simulink model "Flight_sim"  (R2023b)
settings: Solver=ode45  StartTime=0.0  StopTime=350  RelTol=1e-3
values from neighbouring files (symbols this model uses):
  g = 9.81    [parms.m]
  gam_0 = pi/2    (= 1.57079632679)    [parms.m]
  gam_in = 0.10    (= 0.1)    [parms.m]
  h0 = 0    [parms.m]
  m = 132    [parms.m]
  m_zfw = m_dry+m_pay    (= 6360.7)    [parms.m]
  RE = 6371e3    (= 6371000)    [parms.m]
  t_turn = 30    [parms.m]
  v0 = 0.01    [parms.m]
  x0 = 0    [parms.m]
libraries: slpidlib x1, simulink x1
settings Model: Creator=Legrey  LastModifiedBy=Legrey

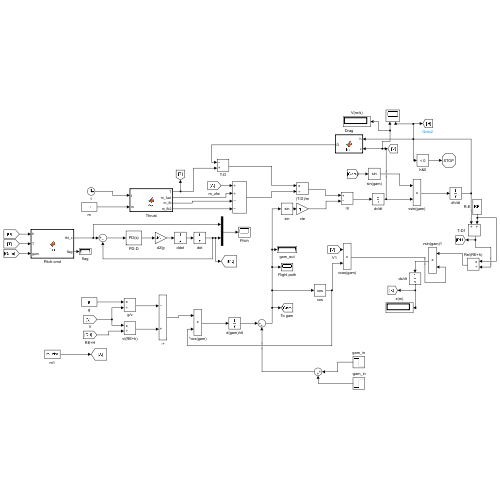
[thumbnail: Simulink's stored preview of the top-level diagram]
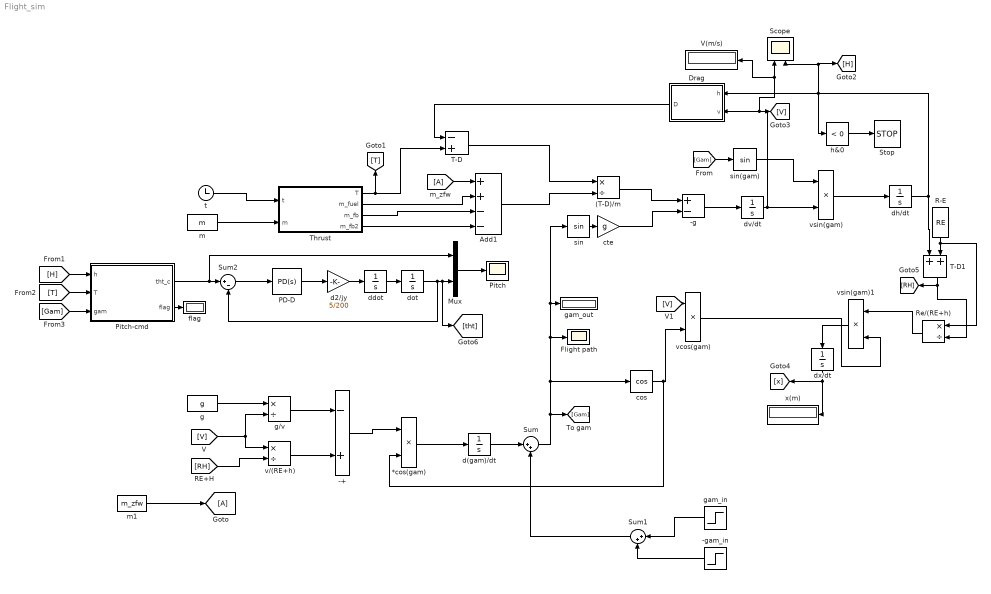
== system Flight_sim ==
  (T-D)/m : Product  Inputs=*/
  *cos(gam) : Product
  -+ : Sum  Inputs=-+
  -g : Sum  Inputs=+-
  -gam_in : Step  Time=t_turn+1  Before=-gam_in  After=-gam_in  SampleTime=0
  Add1 : Sum  Inputs=++--
  Drag : MATLAB Function  TreatAsAtomicUnit=on
  Flight path : Scope
  Goto : Goto
  Mux : Mux  Inputs=2
  PD-D : slpidlib/PID Controller  Controller=PD  Form=Parallel  TimeDomain=Continuous-time  UseExternalTs=off  SampleTime=-1  IntegratorMethod=Forward Euler  FilterMethod=Forward Euler  ControllerParametersSource=internal  P=0  I=1  UseKiTs=off  D=200/5  N=100  UseFilter=on  TunerSelectOption=Transfer Function Based (PID Tuner App)  InitialConditionSource=internal  InitialConditionForIntegrator=0  InitialConditionForFilter=0  DifferentiatorICPrevScaledInput=0  ExternalReset=none  TrackingMode=off  Kt=1  LimitOutput=off  SatLimitsSource=internal  UpperSaturationLimit=inf  LowerSaturationLimit=-inf  LinearizeAsGain=on  AntiWindupMode=none  Kb=1  LimitIntegrator=off  UpperIntegratorSaturationLimit=inf  LowerIntegratorSaturationLimit=-inf  POutMin=[]  POutMax=[]  IOutMin=[]  IOutMax=[]  DOutMin=[]  DOutMax=[]  NOutMin=[]  NOutMax=[]  SumOutMin=[]  SumOutMax=[]  SaturationOutMin=[]  SaturationOutMax=[]  PParamMin=[]  PParamMax=[]  IParamMin=[]  IParamMax=[]  DParamMin=[]  DParamMax=[]  NParamMin=[]  NParamMax=[]  KbParamMin=[]  KbParamMax=[]  KtParamMin=[]  KtParamMax=[]  KbOutMin=[]  KbOutMax=[]  KtOutMin=[]  KtOutMax=[]  IntegratorOutMin=[]  IntegratorOutMax=[]  FilterOutMin=[]  FilterOutMax=[]  SumI1OutMin=[]  SumI1OutMax=[]  SumI2OutMin=[]  SumI2OutMax=[]  SumI3OutMin=[]  SumI3OutMax=[]  SumI4OutMin=[]  SumI4OutMax=[]  SumDOutMin=[]  SumDOutMax=[]  DifferentiatorOutMin=[]  DifferentiatorOutMax=[]  FilterDiffOutCoefMin=[]  FilterDiffOutCoefMax=[]  ReciprocalOutMin=[]  ReciprocalOutMax=[]  SumDenOutMin=[]  SumDenOutMax=[]  SumNumOutMin=[]  SumNumOutMax=[]  DivideOutMin=[]  DivideOutMax=[]  UdiffTsProdOutMin=[]  UdiffTsProdOutMax=[]  NTsProdOutMin=[]  NTsProdOutMax=[]  UintegralTsProdOutMin=[]  UintegralTsProdOutMax=[]  UngainTsProdOutMin=[]  UngainTsProdOutMax=[]  ClampingZeroOutDataTypeStr=Inherit: Inherit via back propagation  ClampingZeroOutMin=[]  ClampingZeroOutMax=[]  FilterDenConstantOutDataTypeStr=Inherit: Inherit via back propagation  FilterDenConstantOutMin=[]  FilterDenConstantOutMax=[]  PCopyOutDataTypeStr=Inherit: Inherit via back propagation  PCopyOutMin=[]  PCopyOutMax=[]  NCopyOutDataTypeStr=Inherit: Inherit via back propagation  NCopyOutMin=[]  NCopyOutMax=[]  IntegratorContinuousStateAttributes=''  IntegratorStateMustResolveToSignalObject=off  IntegratorRTWStateStorageClass=Auto  FilterContinuousStateAttributes=''  FilterStateMustResolveToSignalObject=off  FilterRTWStateStorageClass=Auto  ParallelPVariant=InternalParameters  IdealPVariant=Disabled  IVariant=Disabled  DVariant=InternalParameters  IntegratorVariant=Disabled  SatVariant=Disabled  AWVariant=Disabled  PCopyVariant=Disabled  TRVariant=Disabled  FdbkBlocksVariant=Forward  IdealPFdbkVariant=Disabled  SatFdbkVariant=Disabled  DerivativeFilterVariant=ContFilter  NVariant=InternalParameters  NCopyVariant=Disabled  FilterICVariant=InternalICsFilter  IntegratorICVariant=Disabled  ExternalResetVariant=Disabled  TRSumVariant=Passthrough  SumFdbkVariant=Disabled  SumVariant=Sum_PD  TsampFilterVariant=InternalTs  TsampNgainVariant=Passthrough  TsampIntegralVariant=Disabled_SignalSpec  ExternalSaturationOutDataTypeStr=Inherit: Same as second input
  Pitch : Scope
  Pitch-cmd : MATLAB Function  TreatAsAtomicUnit=on
  R-E : Constant  Value=RE
  Re/(RE+h) : Product  Inputs=*/
  Scope : Scope  NumInputPorts=2
  Stop : Stop
  Sum : Sum  Inputs=|++
  Sum1 : Sum  Inputs=|++
  Sum2 : Sum  Inputs=|+-
  T-D : Sum  Inputs=-+
  T-D1 : Sum
  Thrust : MATLAB Function  TreatAsAtomicUnit=on
  V(m/s) : Display
  cos : Trigonometry  Operator=cos
  cte : Gain  Gain=g
  d(gam)/dt : Integrator  InitialCondition=gam_0
  d2/jy : Gain  Gain=5/200
  ddot : Integrator
  dh/dt : Integrator  InitialCondition=h0
  dot : Integrator  InitialCondition=pi/2
  dv/dt : Integrator  InitialCondition=v0
  dx/dt : Integrator  InitialCondition=x0
  flag : Display
  g : Constant  Value=g
  g/v : Product  Inputs=*/
  gam_in : Step  Time=t_turn  Before=gam_in  After=0  SampleTime=0
  gam_out : Display
  h&0 : simulink/Logic and Bit Operations/Compare To Zero  relop=<  OutDataTypeStr=boolean
  m : Constant  Value=m
  m1 : Constant  Value=m_zfw
  m_zfw : From
  sin : Trigonometry
  sin(gam) : Trigonometry
  t : Clock
  v/(RE+h) : Product  Inputs=*/
  vcos(gam) : Product
  vsin(gam) : Product
  vsin(gam)1 : Product
  x(m) : Display
  wires:
  t/1 -> Thrust/1(t)
  m/1 -> Thrust/2(m)
  Thrust/1(T) -> [T], T-D/2
  Thrust/3(m_fb) -> Add1/3
  Thrust/4(m_fb2) -> Add1/4
  m_zfw/1 -> Add1/1
  m1/1 -> Goto/1
  Thrust/2(m_fuel) -> Add1/2
  T-D/1 -> (T-D)/m/1
  Add1/1 -> (T-D)/m/2
  (T-D)/m/1 -> -g/1
  cte/1 -> -g/2
  sin/1 -> cte/1
  -g/1 -> dv/dt/1
  dv/dt/1 -> V(m/s)/1, Scope/1, [V], Drag/2(v), vsin(gam)/2
  vsin(gam)/1 -> dh/dt/1
  dh/dt/1 -> T-D1/1, Scope/2, [H], h&0/1, Drag/1(h)
  h&0/1 -> Stop/1
  Drag/1(D) -> T-D/1
  R-E/1 -> Re/(RE+h)/1, T-D1/2
  T-D1/1 -> [RH], Re/(RE+h)/2
  Re/(RE+h)/1 -> vsin(gam)1/1
  vsin(gam)1/1 -> dx/dt/1
  dx/dt/1 -> [x], x(m)/1
  g/1 -> g/v/1
  [V] -> v/(RE+h)/1, g/v/2
  [RH] -> v/(RE+h)/2
  g/v/1 -> -+/1
  v/(RE+h)/1 -> -+/2
  -+/1 -> *cos(gam)/1
  *cos(gam)/1 -> d(gam)/dt/1
  d(gam)/dt/1 -> Sum/1
  Sum/1 -> [Gam], cos/1, gam_out/1, sin/1, Flight path/1
  cos/1 -> *cos(gam)/2, vcos(gam)/2
  [V] -> vcos(gam)/1
  vcos(gam)/1 -> vsin(gam)1/2
  [Gam] -> sin(gam)/1
  sin(gam)/1 -> vsin(gam)/1
  gam_in/1 -> Sum1/1
  -gam_in/1 -> Sum1/2
  Sum1/1 -> Sum/2
  [H] -> Pitch-cmd/1(h)
  [T] -> Pitch-cmd/2(T)
  [Gam] -> Pitch-cmd/3(gam)
  Pitch-cmd/2(flag) -> flag/1
  Pitch-cmd/1(tht_c) -> Mux/1, Sum2/1
  Sum2/1 -> PD-D/1
  PD-D/1 -> d2/jy/1
  d2/jy/1 -> ddot/1
  ddot/1 -> dot/1
  dot/1 -> Sum2/2, [tht], Mux/2
  Mux/1 -> Pitch/1

== matlab function Flight_sim/Pitch-cmd ==
  data: h input; tht_c output; T input; gam input; flag output
function [tht_c, flag] = fcn(h, T, gam)

persistent f;
if isempty(f)
     f = 0;
end
if T<=0
    tc = gam+pi;
    if tc>pi
        tc = pi;
    end
    f = 1;
elseif T<=0 && h<1000
    tc = pi/2;
else
    tc = gam;
end
flag = f;
tht_c = tc;

== matlab function Flight_sim/Thrust ==
  data: t input; T output; m_fuel output; m_fb output; m_fb2 output; m input
function [T, m_fuel, m_fb, m_fb2] = fcn(t, m)

persistent mfb;
persistent mfb2;
if isempty(mfb)
    mfb = 0;
end 
if isempty(mfb2)
    mfb2 = 0;
end 
m_fuel = 21491.26;
if mfb <=0.65*m_fuel
    thr = 34691.2;
    mfb = t*m;
else
    thr = 0;
end
if (125<t) && (t<295)
    thr = -110000;
    mfb2 = (t-125)*(m/3);
end
T = thr;
m_fb = mfb;
m_fb2 = mfb2;
m_fuel = mfuel;

== matlab function Flight_sim/Drag ==
  data: h input; D output; v input
function D = fcn(h, v)

CD = 0.075; Di = 1.5; A = pi*Di^2/4; 
%density ISA model:
 if h<=11000 
     T = 15.04 - 0.00649*h; 
     p = 101.29*((T+273.1)/288.08)^5.258;
 elseif (11000<h) && (h<=25000)
    T = -56.46;
    p = 22.65*exp(1.73-0.000157*h);
 else  
     T = -131.21 + 0.00299*h;
     p = 2.488* ((T+273.1)/216.6)^-11.388;
 end 
 rho = p/(0.2869*(T+273.1));
 %drag force D:
 Drag = 0.5*rho*v^2*A*CD; 
 
 D = Drag;
